simulink model "AvoidObstaclesMobileRobot"  (R2021a)
settings: Solver=ode45  StartTime=0.0  StopTime=Inf  RelTol=1e-3
model workspace (MAT data in the model file):
  lidarNoiseSeeds = Simulink.Parameter
  lidarNoiseSeeds.DataType = 'auto'
  lidarNoiseSeeds.Dimensions = [0 0]
undefined symbols (not defined in the file or in its folder): goal_X_max_tolarance, goal_X_min_tolarance, goal_Y_max_tolarance, goal_Y_min_tolarance, goalTheta, goalTheta_max_tolarance, goalTheta_min_tolarance, goalX, goalY, initTheta, initX, initY, mapMatrix, maxAngSpeed, maxLinSpeed, maxRange, min_angle_dis, minimum_lidar_to_wall
libraries: simulink x6, rllib x1, robotmobilelib x1
settings Model: SimulationMode=accelerator  Creator=The MathWorks, Inc.  LastModifiedBy=apizb
settings SolverCC: AlgebraicLoopSolver=TrustRegion
settings OptimizationCC: InitFltsAndDblsToZero=on
settings DebuggingCC: SFMachineParentedDataDiag=warning
settings HardwareCC: ProdLongLongMode=on  TargetLongLongMode=on
settings SFSimCC: SimTargetLang=C++

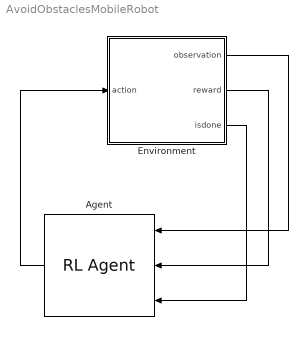
== system AvoidObstaclesMobileRobot ==
  Agent : rllib/RL Agent  Agent=obstacleAvoidanceAgent  ExternalActionAsInput=off  ProvideCumRwd=off  TreatAsDirectFeedthrough=on
      settings: SourceProductName=Reinforcement Learning
  Environment : Subsystem
  wires:
  Environment/1(observation) -> Agent/1
  Environment/2(reward) -> Agent/2
  Environment/3(isdone) -> Agent/3
  Agent/1 -> Environment/1(action)

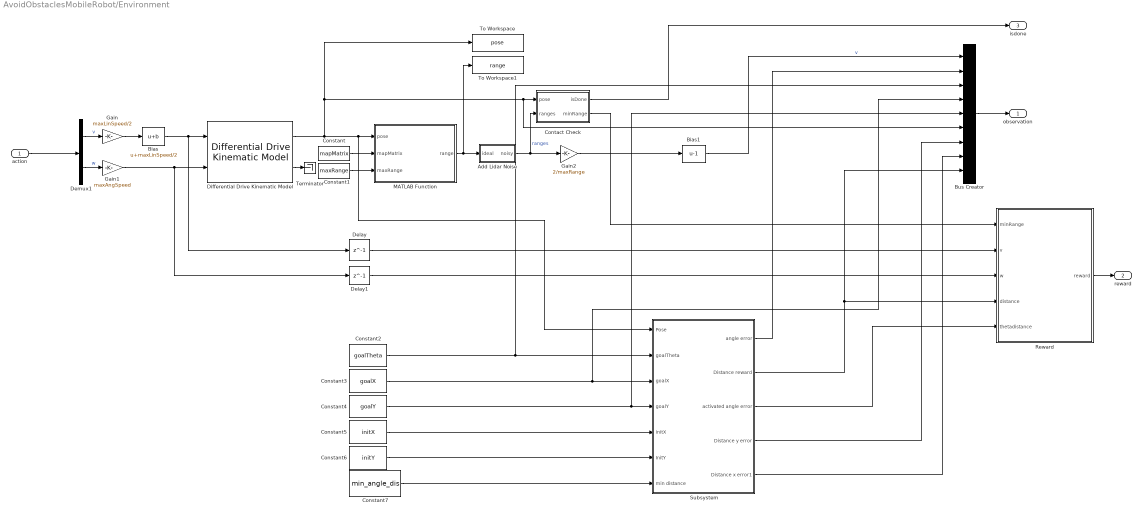
== system AvoidObstaclesMobileRobot/Environment ==
  action : Inport
  Add Lidar Noise : Subsystem
  Bias : Bias  Bias=maxLinSpeed/2
  Bias1 : Bias  Bias=-1
  Bus Creator : BusCreator  Inputs=9
  Constant : Constant  Value=mapMatrix
  Constant1 : Constant  Value=maxRange
  Constant2 : Constant  Value=goalTheta
  Constant3 : Constant  Value=goalX
  Constant4 : Constant  Value=goalY
  Constant5 : Constant  Value=initX
  Constant6 : Constant  Value=initY
  Constant7 : Constant  Value=min_angle_dis
  Contact Check : Subsystem
  Delay : Delay  DelayLength=1  InitialCondition=0  UseCircularBuffer=on
  Delay1 : Delay  DelayLength=1  InitialCondition=0  UseCircularBuffer=on
  Demux1 : Demux  Outputs=2
  Differential Drive Kinematic Model : robotmobilelib/Differential Drive Kinematic Model  VehicleInputs=Vehicle Speed & Heading Angular Velocity  WheelRadius=0.05  WheelSpeedRange=[-inf inf]  TrackWidth=0.2  InitialState=[initX; initY; initTheta]  SimulateUsing=Code generation
      settings: SourceProductName=Robotics System Toolbox
  Gain : Gain  Gain=maxLinSpeed/2
  Gain1 : Gain  Gain=maxAngSpeed
  Gain2 : Gain  Gain=2/maxRange
  MATLAB Function : MATLAB Function  TreatAsAtomicUnit=on
  Reward : Subsystem
  Subsystem : Subsystem
  Terminator : Terminator
  To Workspace : ToWorkspace  VariableName=pose  SampleTime=-1
      settings: Save2DSignal=2-D array (concatenate along first dimension)
  To Workspace1 : ToWorkspace  VariableName=range  SampleTime=-1
  observation : Outport
  reward : Outport  Port=2
  isdone : Outport  Port=3
  wires:
  Differential Drive Kinematic Model/2 -> Terminator/1
  Constant/1 -> MATLAB Function/2(mapMatrix)
  Differential Drive Kinematic Model/1 -> Subsystem/1(Pose), MATLAB Function/1(pose), To Workspace/1, Bus Creator/6, Contact Check/1(pose)
  action/1 -> Demux1/1
  Bias/1 -> Delay/1, Differential Drive Kinematic Model/1
  Gain1/1 -> Delay1/1, Differential Drive Kinematic Model/2
  MATLAB Function/1(range) -> To Workspace1/1, Add Lidar Noise/1(ideal)
  Contact Check/1(isDone) -> isdone/1
  Contact Check/2(minRange) -> Reward/1(minRange)
  Reward/1(reward) -> reward/1
  Gain2/1 -> Bias1/1
  Bias1/1 -> Bus Creator/1  "v"
  Constant1/1 -> MATLAB Function/3(maxRange)
  Delay/1 -> Reward/2(v)
  Delay1/1 -> Reward/3(w)
  Demux1/2 -> Gain1/1  "w"
  Gain/1 -> Bias/1
  Demux1/1 -> Gain/1  "v"
  Add Lidar Noise/1(noisy) -> Gain2/1, Contact Check/2(ranges)  "ranges"
  Subsystem/1(angle error) -> Bus Creator/2
  Bus Creator/1 -> observation/1
  Subsystem/3(activated angle error) -> Reward/5(thetadistance)
  Subsystem/2(Distance reward) -> Bus Creator/9, Reward/4(distance)
  Constant2/1 -> Bus Creator/3, Subsystem/2(goalTheta)
  Constant3/1 -> Bus Creator/4, Subsystem/3(goalX)
  Constant4/1 -> Bus Creator/5, Subsystem/4(goalY)
  Constant5/1 -> Subsystem/5(initX)
  Constant6/1 -> Subsystem/6(InitY)
  Constant7/1 -> Subsystem/7(min distance)
  Subsystem/4(Distance y error) -> Bus Creator/7
  Subsystem/5(Distance x error1) -> Bus Creator/8

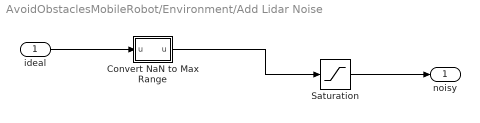
== system AvoidObstaclesMobileRobot/Environment/Add Lidar Noise ==
  ideal : Inport
  Convert NaN to Max Range : MATLAB Function  TreatAsAtomicUnit=on
  Saturation : Saturate  UpperLimit=inf  LowerLimit=0
  noisy : Outport
  wires:
  Convert NaN to Max Range/1(u) -> Saturation/1
  Saturation/1 -> noisy/1
  ideal/1 -> Convert NaN to Max Range/1("u ")

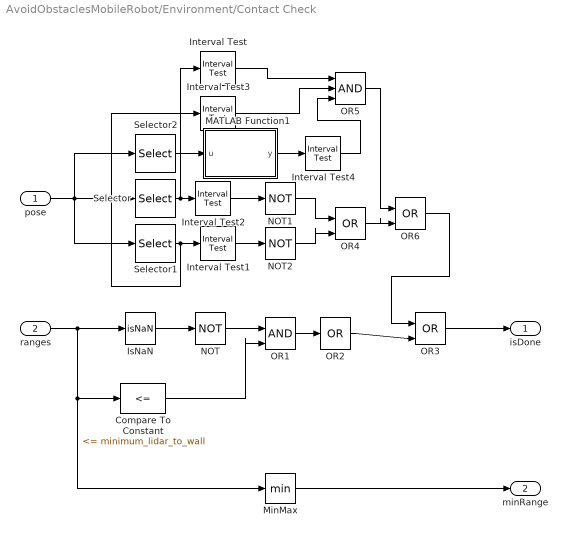
== system AvoidObstaclesMobileRobot/Environment/Contact Check ==
  pose : Inport
  ranges : Inport  Port=2
  Compare To Constant : simulink/Logic and Bit Operations/Compare To Constant  relop=<=  const=minimum_lidar_to_wall  OutDataTypeStr=boolean
  Interval Test : simulink/Logic and Bit Operations/Interval Test  IntervalClosedRight=on  uplimit=goal_X_max_tolarance  IntervalClosedLeft=on  lowlimit=goal_X_min_tolarance  OutDataTypeStr=boolean
  Interval Test1 : simulink/Logic and Bit Operations/Interval Test  IntervalClosedRight=on  uplimit=size(mapMatrix, 1)  IntervalClosedLeft=on  lowlimit=0  OutDataTypeStr=boolean
  Interval Test2 : simulink/Logic and Bit Operations/Interval Test  IntervalClosedRight=on  uplimit=size(mapMatrix, 2)  IntervalClosedLeft=on  lowlimit=0  OutDataTypeStr=boolean
  Interval Test3 : simulink/Logic and Bit Operations/Interval Test  IntervalClosedRight=on  uplimit=goal_Y_max_tolarance  IntervalClosedLeft=on  lowlimit=goal_Y_min_tolarance  OutDataTypeStr=boolean
  Interval Test4 : simulink/Logic and Bit Operations/Interval Test  IntervalClosedRight=on  uplimit=goalTheta_max_tolarance  IntervalClosedLeft=on  lowlimit=goalTheta_min_tolarance  OutDataTypeStr=boolean
  IsNaN : RelationalOperator  Operator=isNaN  OutDataTypeStr=boolean  RndMeth=Simplest
  MATLAB Function1 : MATLAB Function  TreatAsAtomicUnit=on
  MinMax : MinMax
  NOT : Logic  Operator=NOT  IconShape=distinctive  AllPortsSameDT=off  OutDataTypeStr=boolean
  NOT1 : Logic  Operator=NOT  IconShape=distinctive  AllPortsSameDT=off  OutDataTypeStr=boolean
  NOT2 : Logic  Operator=NOT  IconShape=distinctive  AllPortsSameDT=off  OutDataTypeStr=boolean
  OR1 : Logic  IconShape=distinctive  AllPortsSameDT=off  OutDataTypeStr=boolean
  OR2 : Logic  Operator=OR  Inputs=1  IconShape=distinctive  AllPortsSameDT=off  OutDataTypeStr=boolean
  OR3 : Logic  Operator=OR  IconShape=distinctive  AllPortsSameDT=off  OutDataTypeStr=boolean
  OR4 : Logic  Operator=OR  IconShape=distinctive  AllPortsSameDT=off  OutDataTypeStr=boolean
  OR5 : Logic  Inputs=3  IconShape=distinctive  AllPortsSameDT=off  OutDataTypeStr=boolean
  OR6 : Logic  Operator=OR  IconShape=distinctive  AllPortsSameDT=off  OutDataTypeStr=boolean
  Selector : Selector  InputPortWidth=3  IndexOptions=Index vector (dialog)  Indices=1  OutputSizes=1
  Selector1 : Selector  InputPortWidth=3  IndexOptions=Index vector (dialog)  Indices=2  OutputSizes=1
  Selector2 : Selector  InputPortWidth=3  IndexOptions=Index vector (dialog)  Indices=3  OutputSizes=1
  isDone : Outport  VectorParamsAs1DForOutWhenUnconnected=off
  minRange : Outport  Port=2  VectorParamsAs1DForOutWhenUnconnected=off
  wires:
  OR1/1 -> OR2/1
  Compare To Constant/1 -> OR1/2
  NOT/1 -> OR1/1
  ranges/1 -> MinMax/1, Compare To Constant/1, IsNaN/1
  IsNaN/1 -> NOT/1
  MinMax/1 -> minRange/1
  OR3/1 -> isDone/1
  pose/1 -> Selector2/1, Selector/1, Selector1/1
  Selector/1 -> Interval Test/1, Interval Test2/1
  Selector1/1 -> Interval Test3/1, Interval Test1/1
  OR2/1 -> OR3/2
  NOT1/1 -> OR4/1
  Interval Test1/1 -> NOT2/1
  Interval Test2/1 -> NOT1/1
  NOT2/1 -> OR4/2
  Interval Test/1 -> OR5/1
  Interval Test3/1 -> OR5/2
  OR6/1 -> OR3/1
  OR4/1 -> OR6/2
  OR5/1 -> OR6/1
  Interval Test4/1 -> OR5/3
  Selector2/1 -> MATLAB Function1/1(u)
  MATLAB Function1/1(y) -> Interval Test4/1

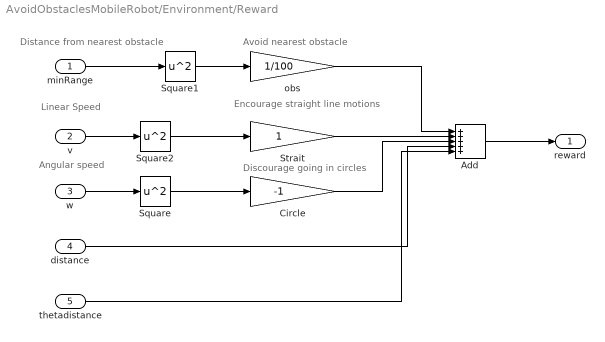
== system AvoidObstaclesMobileRobot/Environment/Reward ==
  note: Discourage going in circles
  note: Encourage straight line motions
  note: Angular speed
  note: Linear Speed
  note: Distance from nearest obstacle
  note: Avoid nearest obstacle
  minRange : Inport
  v : Inport  Port=2
  w : Inport  Port=3
  distance : Inport  Port=4
  thetadistance : Inport  Port=5
  Add : Sum  Inputs=+++++
  Circle : Gain  Gain=-1
  Square : Math  Operator=square  SignedPower=on  SaturateOnIntegerOverflow=on
  Square1 : Math  Operator=square  SignedPower=on  SaturateOnIntegerOverflow=on
  Square2 : Math  Operator=square  SignedPower=on  SaturateOnIntegerOverflow=on
  Strait : Gain
  obs : Gain  Gain=1/100
  reward : Outport  VectorParamsAs1DForOutWhenUnconnected=off
  wires:
  Square/1 -> Circle/1
  w/1 -> Square/1
  Circle/1 -> Add/3
  minRange/1 -> Square1/1
  obs/1 -> Add/1
  Square1/1 -> obs/1
  v/1 -> Square2/1
  Square2/1 -> Strait/1
  Add/1 -> reward/1
  Strait/1 -> Add/2
  thetadistance/1 -> Add/5
  distance/1 -> Add/4

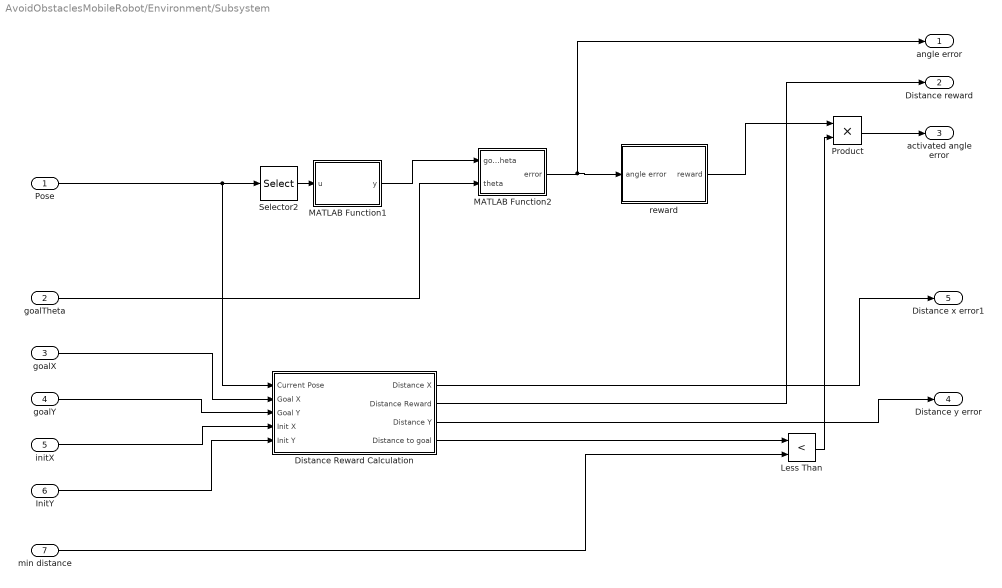
== system AvoidObstaclesMobileRobot/Environment/Subsystem ==
  Pose : Inport
  goalTheta : Inport  Port=2
  goalX : Inport  Port=3
  goalY : Inport  Port=4
  initX : Inport  Port=5
  InitY : Inport  Port=6
  min distance : Inport  Port=7
  Distance Reward Calculation : Subsystem
  Less Than : RelationalOperator  Operator=<  OutDataTypeStr=boolean  RndMeth=Simplest
  MATLAB Function1 : MATLAB Function  TreatAsAtomicUnit=on
  MATLAB Function2 : MATLAB Function  TreatAsAtomicUnit=on
  Product : Product
  Selector2 : Selector  InputPortWidth=3  IndexOptions=Index vector (dialog)  Indices=3  OutputSizes=1
  reward : Subsystem
  angle error : Outport
  Distance reward : Outport  Port=2
  activated angle error : Outport  Port=3
  Distance y error : Outport  Port=4
  Distance x error1 : Outport  Port=5
  wires:
  Pose/1 -> Distance Reward Calculation/1(Current Pose), Selector2/1
  Product/1 -> activated angle error/1
  Less Than/1 -> Product/2
  Selector2/1 -> MATLAB Function1/1(u)
  MATLAB Function2/1(error) -> angle error/1, reward/1(angle error)
  min distance/1 -> Less Than/2
  goalTheta/1 -> MATLAB Function2/2(theta)
  MATLAB Function1/1(y) -> MATLAB Function2/1(goalTheta)
  reward/1(reward) -> Product/1
  Distance Reward Calculation/1(Distance X) -> Distance x error1/1
  Distance Reward Calculation/3(Distance Y) -> Distance y error/1
  goalX/1 -> Distance Reward Calculation/2(Goal X)
  goalY/1 -> Distance Reward Calculation/3(Goal Y)
  initX/1 -> Distance Reward Calculation/4(Init X)
  InitY/1 -> Distance Reward Calculation/5(Init Y)
  Distance Reward Calculation/4(Distance to goal) -> Less Than/1
  Distance Reward Calculation/2(Distance Reward) -> Distance reward/1

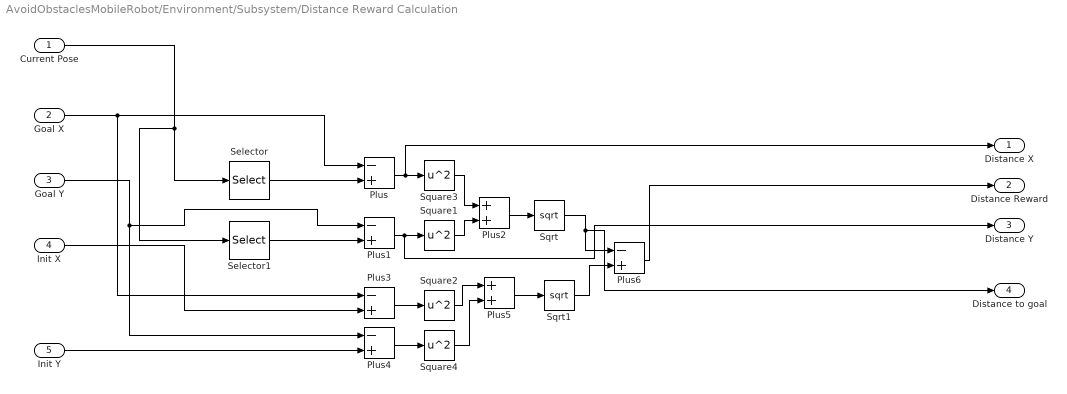
== system AvoidObstaclesMobileRobot/Environment/Subsystem/Distance Reward Calculation ==
  Current Pose : Inport
  Goal X : Inport  Port=2
  Goal Y : Inport  Port=3
  Init X : Inport  Port=4
  Init Y : Inport  Port=5
  Plus{,1,3..4,6} (5 alike) : Sum  Inputs=-+
  Plus2 : Sum
  Plus5 : Sum
  Selector : Selector  InputPortWidth=3  IndexOptions=Index vector (dialog)  Indices=1  OutputSizes=1
  Selector1 : Selector  InputPortWidth=3  IndexOptions=Index vector (dialog)  Indices=2  OutputSizes=1
  Sqrt : Sqrt  SaturateOnIntegerOverflow=on
  Sqrt1 : Sqrt  SaturateOnIntegerOverflow=on
  Square{1..4} (4 alike) : Math  Operator=square  SignedPower=on  SaturateOnIntegerOverflow=on
  Distance X : Outport
  Distance Reward : Outport  Port=2
  Distance Y : Outport  Port=3
  Distance to goal : Outport  Port=4
  wires:
  Plus/1 -> Distance X/1, Square3/1
  Current Pose/1 -> Selector1/1, Selector/1
  Plus4/1 -> Square4/1
  Goal X/1 -> Plus3/1, Plus/1
  Selector1/1 -> Plus1/2
  Plus1/1 -> Distance Y/1, Square1/1
  Sqrt/1 -> Distance to goal/1, Plus6/1
  Square3/1 -> Plus2/1
  Square1/1 -> Plus2/2
  Init Y/1 -> Plus4/2
  Square2/1 -> Plus5/1
  Plus3/1 -> Square2/1
  Selector/1 -> Plus/2
  Square4/1 -> Plus5/2
  Goal Y/1 -> Plus4/1, Plus1/1
  Plus5/1 -> Sqrt1/1
  Plus2/1 -> Sqrt/1
  Sqrt1/1 -> Plus6/2
  Init X/1 -> Plus3/2
  Plus6/1 -> Distance Reward/1

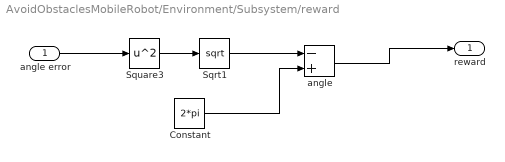
== system AvoidObstaclesMobileRobot/Environment/Subsystem/reward ==
  angle error : Inport
  Constant : Constant  Value=2*pi
  Sqrt1 : Sqrt  SaturateOnIntegerOverflow=on
  Square3 : Math  Operator=square  SignedPower=on  SaturateOnIntegerOverflow=on
  angle : Sum  Inputs=-+
  reward : Outport
  wires:
  angle error/1 -> Square3/1
  Sqrt1/1 -> angle/1
  angle/1 -> reward/1
  Constant/1 -> angle/2
  Square3/1 -> Sqrt1/1

== matlab function AvoidObstaclesMobileRobot/Environment/MATLAB Function ==
  settings: updateMethod=DISCRETE
  data: range output size=[36, 1]; pose input size=[3, 1]; mapMatrix input size=[size(mapMatrix, 1), size(mapMatrix, 2)]; maxRange input; mapScale parameter
function range = RangeSensor(pose, mapMatrix, maxRange, mapScale)
persistent r
if isempty(r)
 r = rangeSensor('HorizontalAngle', [0,2*pi], 'HorizontalAngleResolution', 2*pi/35, 'Range', [0 maxRange]);
end
range = r(pose', binaryOccupancyMap(mapMatrix, mapScale));
end

== matlab function AvoidObstaclesMobileRobot/Environment/Add Lidar Noise/Convert NaN to Max Range ==
  data: u input; u output; maxRange parameter
function u = removeNans(u,maxRange)

u(isnan(u)) = maxRange;

== matlab function AvoidObstaclesMobileRobot/Environment/Subsystem/MATLAB Function1 ==
  data: u input; y output
function y = fcn(u)
x=0;
m=u;
while m<-pi
    m=m+pi;
    %disp('m=');
    %disp(m);
    x=x+1;
    %disp('x=');
    %disp(x);
end
while m>pi
    m=m-pi;
    %disp('m=');
    %disp(m);
    x=x+1;
    %disp('x=');
    %disp(x);
end


% x number you want to know if even or odd
%% create an expression
s = (-1)^x;
%% if s = -1, the N is odd, else N is even
if s == -1
    %disp('x is odd');
    if m>0
        y=m;
    else
        y=m;
    end 
else
    %disp(x);
    %disp('x is even');
    if m>0
        y=m-pi;
    else
        y=m+pi;
    end 
end

== matlab function AvoidObstaclesMobileRobot/Environment/Subsystem/MATLAB Function2 ==
  data: goalTheta input; error output; theta input
function error = fcn2(goalTheta,theta)
if theta>0 && goalTheta>0
    error=goalTheta-theta;
elseif theta>0 && goalTheta<0
    error=-goalTheta+(pi-theta);
elseif theta<0 && goalTheta>0
    error=goalTheta+(pi-theta);
elseif theta<0 && goalTheta<0
    error=goalTheta-theta;
elseif theta==0
    error=goalTheta;
else
    error=0;
end

== matlab function AvoidObstaclesMobileRobot/Environment/Contact Check/MATLAB Function1 ==
  data: u input; y output
function y = fcn(u)
x=0;
m=u;
while m<-pi
    m=m+pi;
    %disp('m=');
    %disp(m);
    x=x+1;
    %disp('x=');
    %disp(x);
end
while m>pi
    m=m-pi;
    %disp('m=');
    %disp(m);
    x=x+1;
    %disp('x=');
    %disp(x);
end


% x number you want to know if even or odd
%% create an expression
s = (-1)^x;
%% if s = -1, the N is odd, else N is even
if s == -1
    %disp('x is odd');
    if m>0
        y=m;
    else
        y=m;
    end 
else
    %disp(x);
    %disp('x is even');
    if m>0
        y=m-pi;
    else
        y=m+pi;
    end 
end
